simulink library "ESTS_VGMG"  (R2024b)
settings: Solver=VariableStepAuto  StartTime=0.0  StopTime=10.0  RelTol=1e-3
undefined symbols (not defined in the file): p_HeiCog_m, p_StatLoaFr_kg, p_StatLoaRe_kg, p_trackFr_m, p_trackRe_m, p_WhlBas_m
settings Model: Creator=blatak  LastModifiedBy=jmbsp
settings ModelReferenceCC: EnableRefExpFcnMdlSchedulingChecks=on
settings RTWCC: GPUComputeCapability=3.5

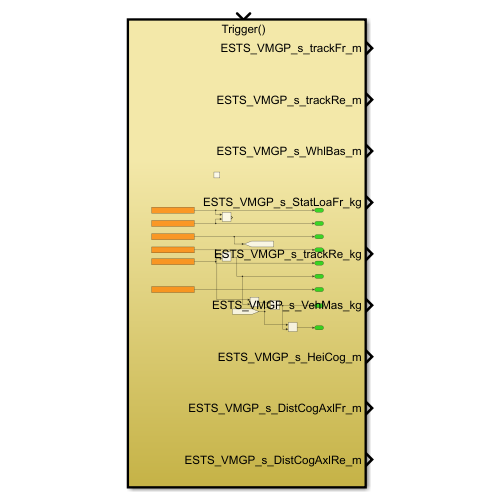
[thumbnail: Simulink's stored preview of the top-level diagram]
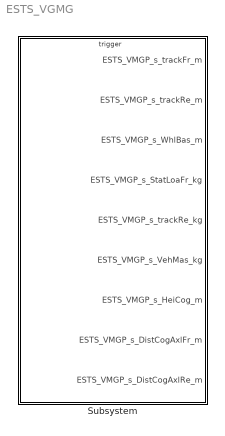
== system ESTS_VGMG ==
  Subsystem : Subsystem

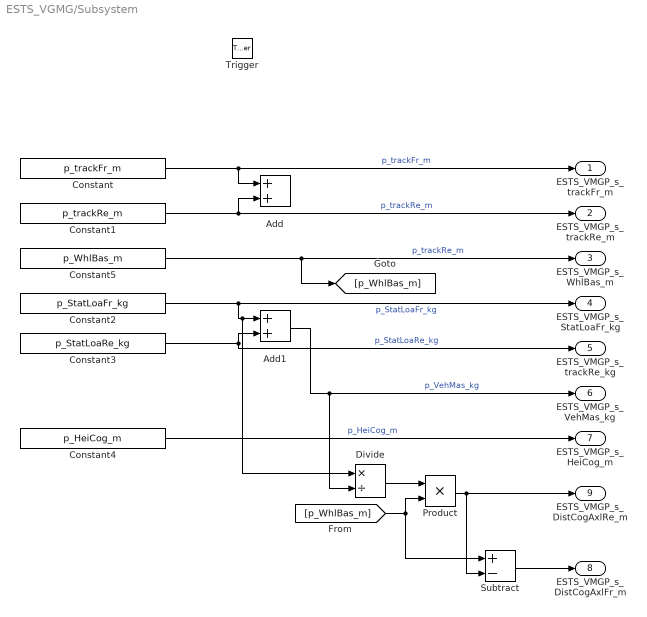
== system ESTS_VGMG/Subsystem ==
  Trigger : TriggerPort  TriggerType=function-call  VariantControl=(inherit)  PortDimensions=1
  Add : Sum
  Add1 : Sum
  Constant : Constant  Value=p_trackFr_m  SampleTime=-1
  Constant1 : Constant  Value=p_trackRe_m  SampleTime=-1
  Constant2 : Constant  Value=p_StatLoaFr_kg  SampleTime=-1
  Constant3 : Constant  Value=p_StatLoaRe_kg  SampleTime=-1
  Constant4 : Constant  Value=p_HeiCog_m  SampleTime=-1
  Constant5 : Constant  Value=p_WhlBas_m  SampleTime=-1
  Divide : Product  Inputs=*/  RndMeth=Zero  SaturateOnIntegerOverflow=on
  Product : Product
  Subtract : Sum  Inputs=+-
  ESTS_VMGP_s_trackFr_m : Outport
  ESTS_VMGP_s_trackRe_m : Outport  Port=2
  ESTS_VMGP_s_WhlBas_m : Outport  Port=3
  ESTS_VMGP_s_StatLoaFr_kg : Outport  Port=4
  ESTS_VMGP_s_trackRe_kg : Outport  Port=5
  ESTS_VMGP_s_VehMas_kg : Outport  Port=6
  ESTS_VMGP_s_HeiCog_m : Outport  Port=7
  ESTS_VMGP_s_DistCogAxlFr_m : Outport  Port=8
  ESTS_VMGP_s_DistCogAxlRe_m : Outport  Port=9
  wires:
  Add1/1 -> Divide/2, ESTS_VMGP_s_VehMas_kg/1  "p_VehMas_kg"
  Constant4/1 -> ESTS_VMGP_s_HeiCog_m/1  "p_HeiCog_m"
  Constant/1 -> Add/1, ESTS_VMGP_s_trackFr_m/1  "p_trackFr_m"
  Constant1/1 -> ESTS_VMGP_s_trackRe_m/1, Add/2  "p_trackRe_m"
  Constant2/1 -> ESTS_VMGP_s_StatLoaFr_kg/1, Divide/1, Add1/1  "p_StatLoaFr_kg"
  Constant3/1 -> ESTS_VMGP_s_trackRe_kg/1, Add1/2  "p_StatLoaRe_kg"
  Divide/1 -> Product/1
  [p_WhlBas_m] -> Product/2, Subtract/1
  Constant5/1 -> [p_WhlBas_m], ESTS_VMGP_s_WhlBas_m/1  "p_trackRe_m"
  Product/1 -> Subtract/2, ESTS_VMGP_s_DistCogAxlRe_m/1
  Subtract/1 -> ESTS_VMGP_s_DistCogAxlFr_m/1
